simulink model "SDmod4"  (R2014b)
settings: Solver=FixedStepDiscrete  SolverMode=SingleTasking  StartTime=0.0  StopTime=(N+Ntransient)*Ts  FixedStep=Ts  MaxStep=3.90625e-06  RelTol=1e-3  AbsTol=1e-3
values from neighbouring files (symbols this model uses):
  Ampl = 0.5    [launch_SDmod4.m]
  finrad = Fin*2*pi    (= 80110.6126665)    [launch_SDmod4.m]
  Fs = OSR*2*bw    (= 6144000)    [launch_SDmod4.m]
  N = 2^13    (= 8192)    [launch_SDmod4.m]
  NCOMPARATORI = 1    [launch_SDmod4.m]
  OSR = 128    [launch_SDmod4.m]
  Ts = 1/Fs    (= 1.62760416667e-07)    [launch_SDmod4.m]
undefined symbols (not defined in the file or in its folder): a, argo, b, c
libraries: SDtoolbox x6
CloseFcn:
  | ;slview('closediagram',bdroot);
settings Model: ExtModeAutoUpdateStatusClock=off  Creator=piero  LastModifiedBy=umi
settings DataIOCC: LimitDataPoints=off  SignalLoggingSaveFormat=ModelDataLogs  SaveOutput=off  SaveTime=off  SignalLoggingName=sigsOut
settings OptimizationCC: BooleanDataType=off  InitFltsAndDblsToZero=on
settings DebuggingCC: SaveWithParameterizedLinksMsg=none  UnderspecifiedInitializationDetection=Classic  MergeDetectMultiDrivingBlocksExec=none  SignalResolutionControl=TryResolveAllWithWarning  SolverPrmCheckMsg=none  MultiTaskDSMMsg=warning  MultiTaskCondExecSysMsg=none  FcnCallInpInsideContextMsg=UseLocalSettings  InitInArrayFormatMsg=none
settings HardwareCC: TargetUnknown=on
settings RTWCC: TemplateMakefile=grt.tmf  IncludeERTFirstTime=on
settings GRTTargetCC: TargetFcnLib=ansi_tfl_tmw.mat  CombineOutputUpdateFcns=off  GRTInterface=on

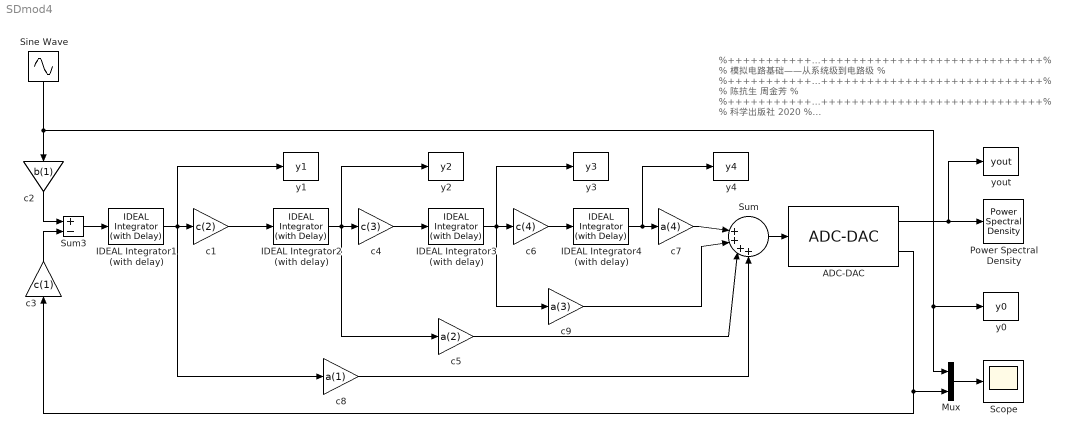
== system SDmod4 ==
  note: %++++++++++++++++++++++++++++++++++++++++%
      | % 模拟电路基础——从系统级到电路级 %
      | %++++++++++++++++++++++++++++++++++++++++%
      | % 陈抗生 周金芳 %
      | %++++++++++++++++++++++++++++++++++++++++%
      | % 科学出版社 2020 %
      | %++++++++++++++++++++++++++++++++++++++++%
  " ADC-DAC" : SDtoolbox/ADC-DAC  k=NCOMPARATORI  MM=off  match=match  CST=Cs  VVG=off  argo=argo(:,3)  LF=off  NF=retA.log
  IDEAL Integrator1 (with delay) : SDtoolbox/IDEAL Integrator (with Delay)  Amax=Amax  Ts=Ts
  IDEAL Integrator2 (with delay) : SDtoolbox/IDEAL Integrator (with Delay)  Amax=Amax  Ts=Ts
  IDEAL Integrator3 (with delay) : SDtoolbox/IDEAL Integrator (with Delay)  Amax=Amax  Ts=Ts
  IDEAL Integrator4 (with delay) : SDtoolbox/IDEAL Integrator (with Delay)  Amax=Amax  Ts=Ts
  Mux : Mux  Inputs=2
  Power Spectral Density : SDtoolbox/Power Spectral Density  SN=7  Fs=Fs  fBL=1  fBH=Fs/(2*OSR)  Fin=Fin  N=N  Ntransient=Ntransient  VW=off  savename=savemat  Scale_type=logarithmic
  Scope : Scope
      settings: YMin=-1  YMax=1  MaxDataPoints=500
  Sine Wave : Sin  Amplitude=Ampl  Frequency=finrad  SampleTime=Ts
  Sum : Sum  Inputs=||++++
  Sum3 : Sum  Inputs=+-  SaturateOnIntegerOverflow=on  InputSameDT=on  OutDataTypeStr=Inherit: Same as first input
  c1 : Gain  Gain=c(2)  SaturateOnIntegerOverflow=on  OutDataTypeStr=Inherit: Same as input  ParamDataTypeStr=Inherit: Same as input
  c2 : Gain  Gain=b(1)  SaturateOnIntegerOverflow=on  OutDataTypeStr=Inherit: Same as input  ParamDataTypeStr=Inherit: Same as input
  c3 : Gain  Gain=c(1)  SaturateOnIntegerOverflow=on  OutDataTypeStr=Inherit: Same as input  ParamDataTypeStr=Inherit: Same as input
  c4 : Gain  Gain=c(3)  SaturateOnIntegerOverflow=on  OutDataTypeStr=Inherit: Same as input  ParamDataTypeStr=Inherit: Same as input
  c5 : Gain  Gain=a(2)  SaturateOnIntegerOverflow=on  OutDataTypeStr=Inherit: Same as input  ParamDataTypeStr=Inherit: Same as input
  c6 : Gain  Gain=c(4)  SaturateOnIntegerOverflow=on  OutDataTypeStr=Inherit: Same as input  ParamDataTypeStr=Inherit: Same as input
  c7 : Gain  Gain=a(4)  SaturateOnIntegerOverflow=on  OutDataTypeStr=Inherit: Same as input  ParamDataTypeStr=Inherit: Same as input
  c8 : Gain  Gain=a(1)  SaturateOnIntegerOverflow=on  OutDataTypeStr=Inherit: Same as input  ParamDataTypeStr=Inherit: Same as input
  c9 : Gain  Gain=a(3)  SaturateOnIntegerOverflow=on  OutDataTypeStr=Inherit: Same as input  ParamDataTypeStr=Inherit: Same as input
  y0 : ToWorkspace  VariableName=y0  SampleTime=-1
  y1 : ToWorkspace  VariableName=y1  SampleTime=-1
  y2 : ToWorkspace  VariableName=y2  SampleTime=-1
  y3 : ToWorkspace  VariableName=y3  SampleTime=-1
  y4 : ToWorkspace  VariableName=y4  SampleTime=-1
  yout : ToWorkspace  VariableName=yout  SampleTime=-1
  wires:
  c1/1 -> IDEAL Integrator2 (with delay)/1
  Sine Wave/1 -> y0/1, Mux/1, c2/1
  " ADC-DAC"/1 -> yout/1, Power Spectral Density/1
  IDEAL Integrator2 (with delay)/1 -> y2/1, c5/1, c4/1
  c2/1 -> Sum3/1
  c3/1 -> Sum3/2
  " ADC-DAC"/2 -> c3/1, Mux/2
  Sum3/1 -> IDEAL Integrator1 (with delay)/1
  IDEAL Integrator1 (with delay)/1 -> c1/1, y1/1, c8/1
  Mux/1 -> Scope/1
  c4/1 -> IDEAL Integrator3 (with delay)/1
  IDEAL Integrator3 (with delay)/1 -> y3/1, c9/1, c6/1
  IDEAL Integrator4 (with delay)/1 -> y4/1, c7/1
  c6/1 -> IDEAL Integrator4 (with delay)/1
  c7/1 -> Sum/1
  c8/1 -> Sum/4
  c5/1 -> Sum/3
  c9/1 -> Sum/2
  Sum/1 -> " ADC-DAC"/1
